simulink model "timer_simulink_example"  (R2021b)
settings: Solver=FixedStepAuto  StartTime=0.0  StopTime=inf  FixedStep=0.01  RelTol=1e-3
libraries: stimer_slib x4
settings Model: Creator=LCD  LastModifiedBy=Camilo
settings SolverCC: AlgebraicLoopSolver=TrustRegion
settings DebuggingCC: SFMachineParentedDataDiag=warning

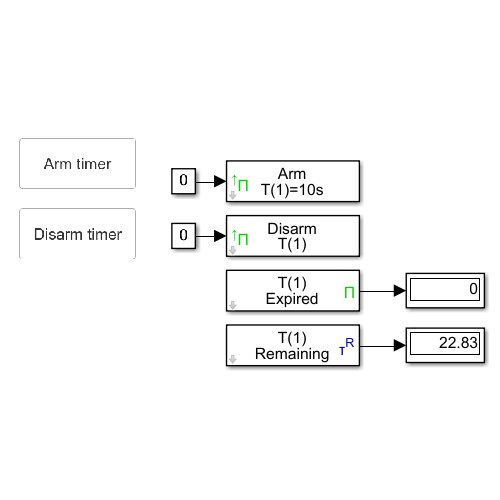
[thumbnail: Simulink's stored preview of the top-level diagram]
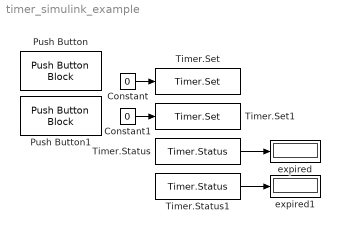
== system timer_simulink_example ==
  Constant : Constant  Value=0
  Constant1 : Constant  Value=0
  Push Button : PushButtonBlock  ButtonText=Arm timer  OffValue=0.000000
  Push Button1 : PushButtonBlock  ButtonText=Disarm timer  OffValue=0.000000
  Timer.Set : stimer_slib/Timer.Set  tindex=1  tvalue=10
      settings: SourceProductName=STimer
  Timer.Set1 : stimer_slib/Timer.Set  tindex=1  tvalue=0
      settings: SourceProductName=STimer
  Timer.Status : stimer_slib/Timer.Status  xtimer=1  prop=Expired
      settings: SourceProductName=STimer
  Timer.Status1 : stimer_slib/Timer.Status  xtimer=1  prop=Remaining
      settings: SourceProductName=STimer
  expired : Display
  expired1 : Display
  wires:
  Constant/1 -> Timer.Set/1
  Constant1/1 -> Timer.Set1/1
  Timer.Status/1 -> expired/1
  Timer.Status1/1 -> expired1/1
